simulink model "UNCCModel"  (R2018b)
settings: Solver=ode4  StartTime=0.0  StopTime=Inf  FixedStep=0.025  RelTol=1e-3  EnableMultiTasking=on
PreLoadFcn:
  | preLoadCallback
StartFcn:
  | startCallback
StopFcn:
  | stopCallback
model workspace (MAT data in the model file):
  Ts = 0.025
undefined symbols (not defined in the file or in its folder): acA2000, Ace, Basler, Freerun_FIX_YAW, PoCL
libraries: slrtlib x3, xpcbitflowlib x3, xpcvideoutillib x2, xpcobsoletelib x1, xpcrtudplib x1
(part 3 of 3)

== matlab function UNCCModel/cam3A/convertPixelsToCM ==
  data: d input; xx output; yx output; xTop input; xBottom input; yTop input; yBottom input; viewAngle input
function [xx,yx] = ...
    convertPixelsToLength(d,xTop,xBottom,yTop,yBottom,viewAngle)
%#codegen

% INPUTS:
% d - distance from camera to dot centroid
% xTop - horizontal pixel coordinate location of left dot in the frame
% xBottom - horizontal pixel coordinate location of the right dot in the
% frame
% yTop - vertical pixel coordinate location of the left dot in the frame
% yBottom -  vertical pixel coordinate location of the right dot in the
% frame
% viewAngle - two element vector, first characterizes the width of the
% field of view (camera horizontal), the second characterizes the height of
% the field of veiw (camera vertical).

% Calculate dot separations in pixels
% Camera-X separation will contribute to y component of body fixed x unit
% vector, if top dot is to the left of bottom dot (xTop<xBottom), then the component will
% have a negative value.  Camera-Y separation will contribute to x 
% component of body fixed x unit vector if top dot is above bottom dot 
% (yTop<yBottom), then this should have a positive value.  Note that 
% coordinate origin of pixels is in the upper left of the frame and the 
% positive y points down.
xx = -(yTop - yBottom);
yx =  (xTop - xBottom); 


% Convert pixels to length
% The (2*d*tand(viewAngle(1))) term calculates the total horizontal (or
% vertical)
% distance spanned by the camera field of view, the /2040 and /1080 terms
% normalize the separations by the total number of pixels.
xx = (2*d*tand(viewAngle(2)))*(xx/1088);
yx = (2*d*tand(viewAngle(1)))*(yx/2040);


xc=(yTop+yBottom)/2;
yc=(xTop+xBottom)/2;
xx = xx/cosd(20*((544-xc)/544));
yx = yx/cosd(20*((1020-yc)/1020));

== matlab function UNCCModel/cam2/convertPixelsToCM ==
  data: d input; yy output; zy output; xLeft input; xRight input; yLeft input; yRight input; viewAngle input
function [yy, zy] = ...
    convertPixelsToLength(d,xLeft,xRight,yLeft,yRight,viewAngle)
%#codegen

% INPUTS:
% d - distance from camera to dot centroid
% xLeft - horizontal pixel coordinate location of left dot in the frame
% xRight - horizontal pixel coordinate location of the right dot in the
% frame
% yLeft - vertical pixel coordinate location of the left dot in the frame
% yRight -  vertical pixel coordinate location of the right dot in the
% frame
% viewAngle - two element vector, first characterizes the width of the
% field of view (camera horizontal), the second characterizes the height of
% the field of veiw (camera vertical).

% Calculate dot separations in pixels
% Camera-X separation will contribute to y component of body fixed y unit
% vector, if left dot is to the left of right dot (xLeft<xRight), then the 
% component will have a positive value.  Camera-Y separation
% will contribute to z component of body fixed y unit vector if left dot is
% below right dot (yLeft>yRight),
% then this should have a positive value.
yy = -(xLeft - xRight); 
zy =  (yLeft - yRight);

% Convert pixels to length
% The (2*d*tand(viewAngle(1))) term calculates the total horizontal (or
% vertical)
% distance spanned by the camera field of view, the /2040 and /1080 terms
% normalize the separations by the total number of pixels.
yy = (2*d*tand(viewAngle(1)))*(yy/2040); % y component of body fixed y
zy = (2*d*tand(viewAngle(2)))*(zy/1088); % z component of body fixed y


yc=(xLeft+xRight)/2;
zc=(yLeft+yRight)/2;
yy = yy/cosd(20*((544-yc)/544));
zy = zy/cosd(20*((1020-zc)/1020));

== matlab function UNCCModel/cam3B/convertPixelsToCM ==
  data: d input; xy output; yy output; xLeft input; xRight input; yLeft input; yRight input; viewAngle input
function [xy, yy] = ...
    convertPixelsToLength(d,xLeft,xRight,yLeft,yRight,viewAngle)
%#codegen

% INPUTS:
% d - distance from camera to dot centroid
% xLeft - horizontal pixel coordinate location of left dot in the frame
% xRight - horizontal pixel coordinate location of the right dot in the
% frame
% yLeft - vertical pixel coordinate location of the left dot in the frame
% yRight -  vertical pixel coordinate location of the right dot in the
% frame
% viewAngle - two element vector, first characterizes the width of the
% field of view (camera horizontal), the second characterizes the height of
% the field of veiw (camera vertical).

% Calculate dot separations in pixels
% Camera-X separation will contribute to y component of body fixed y unit
% vector, if left dot is to the left of right dot (xLeft<xRight), then the 
% component will have a positive value.  Camera-Y separation
% will contribute to x component of body fixed y unit vector if left dot is
% below right dot (yLeft>yRight),
% then this should have a positive value.
yy = -(xLeft - xRight); 
xy =  (yLeft - yRight);

% Convert pixels to length
% The (2*d*tand(viewAngle(1))) term calculates the total horizontal (or
% vertical)
% distance spanned by the camera field of view, the /2040 and /1080 terms
% normalize the separations by the total number of pixels.
xy = (2*d*tand(viewAngle(1)))*(xy/2040); % y component of body fixed y
yy = (2*d*tand(viewAngle(2)))*(yy/1080); % z component of body fixed y


yc=(xLeft+xRight)/2;
xc=(yLeft+yRight)/2;
yy = yy/cosd(20*((544-yc)/544));
xy = xy/cosd(20*((1020-xc)/1020));

== matlab function UNCCModel/cam3A/convertAbsolutePositionToCM ==
  data: rCam input; xCam input; yCam input; viewAngle input; d input; r output
function r = convertAbsolutePositionsToCM(rCam, xCam, yCam,  viewAngle, d)
%#codegen
% This function calculates the x, y and z position of the dots in the
% ground fixed coordinates

% INPUTS
% rCam - 3 element vector of the camera position in the ground fixed frame
% units:cm
% xCam - horitontal location of the dots centroid in the image frame
% units:pixels
% yCam - vertical location of the dots centroid in the image frame
% units:pixels
% viewAngle - two element vector, first characterizes the width of the
% field of view (camera horizontal), the second characterizes the height of
% the field of veiw (camera vertical).
% d - distance from the camera to the dots

% Calculate the x and y locations
% If the horizontal location of the dots centroid in the image frame is
% to the left of the centerline (xCam<1020) then the y position of the dots
% centroid in the ground fixed frame will be greater than the y position of
% the camera in the ground fixed frame.
% If the vertical location of the dots centroid in the image frame is
% below the centerline (yCam>544) then the x position of the dots
% centroid in the ground fixed frame will be greater than the x position of
% the camera in the ground fixed frame.
% d=50;
x = rCam(1) + (yCam - 544 )*((2*d*tand(viewAngle(1)))/1088);
y = rCam(2) - (xCam - 1020)*((2*d*tand(viewAngle(2)))/2040);

% Calculate the z coordinate of the centroid of the dots.
% We know the x and y coordinate, the position of the camera, and the
% distance fromt the cammera to the dots.  Therfore, the solution is the
% value of z which causes the position to lie on the sphere centered on the
% camera with radius = d
z = 0;
% Check first to make sure that the value under the sqrt is positive
if d^2-(x - rCam(1))^2-(y - rCam(2))^2>=0
    z  = rCam(3) + sqrt(d^2-(x - rCam(1))^2-(y - rCam(2))^2);
end

r  =  [x y z];

== matlab function UNCCModel/cam3B/convertAbsolutePositionToCM ==
  data: rCam input; xCam input; yCam input; viewAngle input; d input; r output
function r = convertAbsolutePositionsToCM(rCam, xCam, yCam,  viewAngle, d)
%#codegen
% This function calculates the x, y and z position of the dots in the
% ground fixed coordinates

% INPUTS
% rCam - 3 element vector of the camera position in the ground fixed frame
% units:cm
% xCam - horitontal location of the dots centroid in the image frame
% units:pixels
% yCam - vertical location of the dots centroid in the image frame
% units:pixels
% viewAngle - two element vector, first characterizes the width of the
% field of view (camera horizontal), the second characterizes the height of
% the field of veiw (camera vertical).
% d - distance from the camera to the dots

% Calculate the x and y locations
% If the horizontal location of the dots centroid in the image frame is
% to the left of the centerline (xCam<1020) then the y position of the dots
% centroid in the ground fixed frame will be less than the y position of
% the camera in the ground fixed frame.
% If the vertical location of the dots centroid in the image frame is
% below the centerline (yCam>544) then the x position of the dots
% centroid in the ground fixed frame will be greater than the x position of
% the camera in the ground fixed frame.
% d=50;
x = rCam(1) + (yCam - 544 )*((2*d*tand(viewAngle(1)))/1088);
y = rCam(2) + (xCam - 1020)*((2*d*tand(viewAngle(2)))/2040);

% Calculate the z coordinate of the centroid of the dots.
% We know the x and y coordinate, the position of the camera, and the
% distance fromt the cammera to the dots.  Therfore, the solution is the
% value of z which causes the position to lie on the sphere centered on the
% camera with radius = d
z = 0;
% Check first to make sure that the value under the sqrt is positive
if d^2-(x - rCam(1))^2-(y - rCam(2))^2>=0
    z  = rCam(3) + sqrt(d^2-(x - rCam(1))^2-(y - rCam(2))^2);
end

r  =  [x y z];

== matlab function UNCCModel/MATLAB Function1 ==
  data: errorFlag input; controlMode input; motorVoltages output; closedLoopMotorCommands input; GUIMotorCommands input; saturation input
function motorVoltages = fcn(errorFlag,controlMode, closedLoopMotorCommands, GUIMotorCommands,saturation)
%#codegen

motorVoltages = GUIMotorCommands*1.65;
if controlMode == 1 % control mode 1 is closed loop control
    motorVoltages = closedLoopMotorCommands;
    
end

motorVoltages = motorVoltages + 1.65; %apply constant offset

if errorFlag ==1 % if there's a NaN error, zero all motors
    motorVoltages = 1.65*[1 1 1]';
    
end
for i = 1:3
    if motorVoltages(i)>saturation
        motorVoltages(i)=saturation;
    end
end

end

== matlab function UNCCModel/pitchDeadband ==
  data: onOff input; thetaSP input; theta input; error output; DBUpperLim input; DBLowerLim input
function error = fcn(onOff,thetaSP,theta,DBUpperLim,DBLowerLim)
%#codegen
error = 0;
if onOff == 1 % if onOff = 1, turn on the deadband
    if theta < thetaSP + DBLowerLim
        error = DBLowerLim - theta;
    end
    
    if theta > thetaSP + DBUpperLim
        error = DBUpperLim - theta;
    end
else % if onOff !=0 then turn off the deadband and use normal error
    error = thetaSP-theta;
end
end

== matlab function UNCCModel/cam1/Dot_detector_pitch ==
  data: uOut output; u input; roiDims input; locationMethod input; dotConfig input; centroidOverrideCommand input; rCentroidManualOverride input; clusteringParameters input; rCentroidAuto input; r1Img output; r2Img output; rCentroidImg output; viewOptions input
function [uOut,r1Img,r2Img,rCentroidImg] =...
    dotFinder(u,roiDims, locationMethod, dotConfig,centroidOverrideCommand,rCentroidManualOverride,clusteringParameters,rCentroidAuto,viewOptions)
%#codegen
% EXPLANATION OF INPUTS
% u = source image
% roiDims = 4 by 1 vector containing ROI dimensions
% locationMethod = 0 for centroid based dot location
% locationMethod = 1 for cluster based dot location (longer runtime but
% more robust
% dotConfig = 0 for horizontally arranged dots
% dotConfig = 1 for vertically arranged dots
% centroidOverrideCommand = 0 for automatic movemennt of ROI
% centroidOverrideCommand = 1 to use user input as ROI location
% rCentroidManualOverride: 2 element vector where element 1 is x or column
% of ROI centroid and element 2 is y or row of ROI, both of which are
% manually enetered by used
% rCentroidAuto: 2 element vector where element 1 is x or column of ROI
% centroid and element 2 is y or row of ROI, both of which are
% automatically generated from previous iteration
% viewOptions : 8 element vector where each element is a binary on/off
% switch to a certain part of the output view window
%
% WHAT THIS CODE IS
% Method : Centroid Only
%
% This code is a first attempt at rewriting the code to allow for adaptable
% implemmentation.
% Adaptable implemmentation will ultimately include:
% switch to change between DB clustering and centroid method
%



%%%%%%%%%%%%%%%%%%%%
% SET ROI DIMENSIONS
%%%%%%%%%%%%%%%%%%%%
[ roiHalfwidth, roiHalfheight ] = getROIDimensions(dotConfig,roiDims,centroidOverrideCommand);

%%%%%%%%%%%%%%%%%%%%
% PARSE INPUTS
%%%%%%%%%%%%%%%%%%%%

[dotConfig, locationMethod, centroidOverrideCommand ,rCentroidManualOverride ,viewOptions,roiHalfwidth, roiHalfheight]...
    =parseInputs(dotConfig, locationMethod, centroidOverrideCommand ,rCentroidManualOverride ,viewOptions,roiHalfwidth, roiHalfheight);

%%%%%%%%%%%%%%%%%%%%
%%SET ROI LOCATION%%
%%%%%%%%%%%%%%%%%%%%
rCentroid = rCentroidAuto;
if centroidOverrideCommand == 1  %Override with user input if commanded to do so
    rCentroid = rCentroidManualOverride;
end

%%%%%%%%%%%%%%%%%%%%%%%%%%%%%%%%%%%%
% EXTRACT ROI FROM ORIGIONAL IMAGE %
%%%%%%%%%%%%%%%%%%%%%%%%%%%%%%%%%%%%
roi=u(rCentroid(2) - roiHalfheight : rCentroid(2) + roiHalfheight , rCentroid(1) - roiHalfwidth : rCentroid(1) + roiHalfwidth);

%%%%%%%%%%%%%%%%%%%%%%%%%%%%%
%%%%OTSUS METHOD THRESHOLDING
%%%%%%%%%%%%%%%%%%%%%%%%%%%%%
roi=threshold(roi);


%%%%%%%%%%%%%%%%
% DOT LOCATION %
%%%%%%%%%%%%%%%%
%Preallocate to avoid "Variable undefined on some iteration paths" compile
%error
r1ROI        = [0,0]; r2ROI        = [0,0]; rCentroidROI = [0,0];
if locationMethod == 0; %USE CENTROID BASED METHOD
    if dotConfig == 0 %%HORIZONTAL DOTS
        [r1ROI,r2ROI,rCentroidROI] = centroidMethodHorizontal(roi,roiHalfwidth,roiHalfheight);
    else                %%VERTICAL DOTS
        [r1ROI,r2ROI,rCentroidROI] = centroidMethodVertical(roi,roiHalfwidth,roiHalfheight);
    end
else %USE CLUSTERING BASED METHOD (NOT CURRENTLY IMPLEMENTED)
    %%%REPLACE THIS CODE WITH CLUSTERING METHOD WHEN IMPLEMENTING
    %%%UNCOMMENT CODE BELOW ONCE clusterMethod FUNCTION IS WRITTEN
    %%%[r1ROI,r2ROI,rCentroidROI] = clusterMethod(roi,clusteringParameters);
    if dotConfig == 0 %%HORIZONTAL DOTS
        [r1ROI,r2ROI,rCentroidROI] = centroidMethodHorizontal(roi,roiHalfwidth,roiHalfheight);
    else                %%VERTICAL DOTS
        [r1ROI,r2ROI,rCentroidROI] = centroidMethodVertical(roi,roiHalfwidth,roiHalfheight);
    end
end
%%%%%%%%%%%%%%%%%%%%%%%%%
%%%%PARSE DOT LOCATIONS %
%%%%%%%%%%%%%%%%%%%%%%%%%
%IF DOT CENTER LOCATION ALGORITHM HAS FAILED (OUTPUT = NONSENSE) THEN
%OVERRIDE CENTROID COORDINATES WITH DEFAULT VALUES TO PREVENT PROBLEMS
%LATER
[r1ROI,r2ROI,rCentroidROI] = parseDotLocations(dotConfig,r1ROI,r2ROI,rCentroidROI,roiHalfwidth,roiHalfheight);

%%%%%%%%%%%%%%%%%%%%%%%%%%%%%%%%%%%%%%%%%%%%%%%%%%%
%%%%TRANSFORM BACK TO ORIGIONAL IMAGE COORDINATES %
%%%%%%%%%%%%%%%%%%%%%%%%%%%%%%%%%%%%%%%%%%%%%%%%%%%
%Preallocate to avoid "Variable undefined on some iteration paths" compile
%error
r1Img         = [0,0]; r2Img         = [0,0]; rCenntroidImg = [0,0];

if dotConfig == 0  %HORIZONTALLY ARRANGED DOTS
    [r1Img, r2Img, rCentroidImg] = convertCoordinatesHorizontal(r1ROI,r2ROI,rCentroid,roiHalfwidth,roiHalfheight);
else % VERTICALLY ARRANGED DOTS
    [r1Img, r2Img, rCentroidImg] = convertCoordinatesVertical(r1ROI,r2ROI,rCentroid,roiHalfwidth,roiHalfheight);
end
%%%%%%%%%%%%%%%%%%%%%
% DRAW OUTPUT IMAGE %
%%%%%%%%%%%%%%%%%%%%%

uOut  =  drawOutputImage(viewOptions,u,roi,r1Img,r2Img,rCentroid,r1ROI,r2ROI,roiHalfwidth,roiHalfheight);


end



%DRAW OUTPUT IMAGE
function uOut  =  drawOutputImage(viewOptions,uOut,roi,r1Img,r2Img,rCentroid,r1ROI,r2ROI,roiHalfwidth,roiHalfheight)
%function takes the origional image "u" and redraws it as the output image
%uOut
%View options 7 and 8 are currently not used, can/will be used later for
%clustering algorithm outputs
if viewOptions(1) == 1 %View option = draw any features on output view at all
    if viewOptions(2) == 1 %Draw Features in main image
        if viewOptions(3) == 1 %Draw ROI box in main image
            uOut(rCentroid(2) - roiHalfheight : rCentroid(2) + roiHalfheight, rCentroid(1) - roiHalfwidth                               )=255; %Draw left edge of roi box
            uOut(rCentroid(2) - roiHalfheight : rCentroid(2) + roiHalfheight, rCentroid(1) + roiHalfwidth                               )=255; %Draw right edge of roi box
            uOut(rCentroid(2) - roiHalfheight                               , rCentroid(1) - roiHalfwidth : rCentroid(1)+roiHalfwidth  )=255; %Draw top edge of roi box
            uOut(rCentroid(2) + roiHalfheight                               , rCentroid(1) - roiHalfwidth : rCentroid(1)+roiHalfwidth  )=255; %Draw bottom edge of roi box
        end
        if viewOptions(4) == 1 %Draw crosshairs in main image
            uOut(: ,r1Img(1)  ) = 255;
            uOut(: ,r2Img(1) ) = 255;
            uOut(r1Img(2) ,:  ) = 255;
            uOut(r2Img(2),:  ) = 255;
        end
    end
    if viewOptions(5) == 1 %Draw thresholding in lower left
        roi = 255*roi;
        if viewOptions(6) == 1% Draw crosshairs on thresholding
            roi(r1ROI(2) , :           ) = 255;
            roi(r2ROI(2), :           ) = 255;
            roi(:           , r1ROI(1) ) = 255;
            roi(:           , r2ROI(1)) = 255;
        end
        uOut (1080-size(roi,1)+1:1080, 1:size(roi,2)) = roi;
    end
end
end

%CONVERT ROI COORDINATES TO IMG COORDINATES (HORIZONTAL)
function [rLeftImg, rRightImg, rCentroidImg] = convertCoordinatesHorizontal(rLeftROI,rRightROI,rCentroid,roiHalfwidth,roiHalfheight)
%This function takes in the dot positions in the ROI frame of reference
%and outputs coordinates in the origional image frame of reference, all in
%vectorize format [x,y].  Note that x = column and y = row.

%Convert y (row) coordinates
yLImg = rCentroid(2) - roiHalfheight + rLeftROI(2);
yRImg = rCentroid(2) - roiHalfheight + rRightROI(2);
%Convert x (col) coordinates
xLImg = rCentroid(1) - roiHalfwidth + rLeftROI(1);
xRImg = rCentroid(1) - roiHalfwidth + rRightROI(1);
%Put results into vector format
rLeftImg  = [ xLImg, yLImg ];
rRightImg = [ xRImg, yRImg ];
%Calculate ROI cenntroid as average of two dot coordinates
rCentroidImg = [fix((xLImg+xRImg)/2),fix((yLImg+yRImg)/2)];

end

%CONVERT ROI COORDINATES TO IMG COORDINATES (VERTICAL)
function [rTopImg, rBottomImg, rCentroidImg] = convertCoordinatesVertical(rTopROI,rBottomROI,rCentroid,roiHalfwidth,roiHalfheight)
%This function takes in the dot positions in the ROI frame of reference
%and outputs coordinates in the origional image frame of reference, all in
%vectorize format [x,y].  Note that x = column and y = row.

%Convert y (row) coordinates
yTImg = rCentroid(2) - roiHalfheight + rTopROI(2);
yBImg = rCentroid(2) - roiHalfheight + rBottomROI(2);
%Convert x (col) coordinates
xTImg = rCentroid(1) - roiHalfwidth + rTopROI(1);
xBImg = rCentroid(1) - roiHalfwidth + rBottomROI(1);
%Put results into vector format
rTopImg    = [ xTImg, yTImg ];
rBottomImg = [ xBImg, yBImg ];
%Calculate ROI cenntroid as average of two dot coordinates
rCentroidImg = [fix((xTImg+xBImg)/2),fix((yTImg+yBImg)/2)];

end

%CENTROID METHOD DOT LOCATION (HORIZONTAL)
function [rLeft,rRight,rCentroid] = centroidMethodHorizontal(roi,roiHalfwidth,roiHalfheight)
%Function returns the position of the dots rCentroid as well as the
%centroid of the overall image rCentroid
%Calculated by using centroid method, assuming the dots are arranged
%horizontally

%Divide the image in half vertically (left and right)
roiLeft  = roi( : , 1            : roiHalfwidth);
roiRight = roi( : , roiHalfwidth : end         );

%Calculate the x coordinates of the centroids
xLROI = round(sum((sum(roiLeft ,1) .* (1:size(roiLeft ,2))))/sum(sum(roiLeft )));
xRROI = round(sum((sum(roiRight,1) .* (1:size(roiRight,2))))/sum(sum(roiRight)))+roiHalfwidth;
%Calculate the y coordinates of the centroids
yLROI = round(sum((sum(roiLeft ,2) .* (1:size(roiLeft, 1))'))/sum(sum(roiLeft )));
yRROI = round(sum((sum(roiRight,2) .* (1:size(roiRight,1))'))/sum(sum(roiRight)));
%Put results into vector format
rLeft     = [xLROI, yLROI];
rRight    = [xRROI, yRROI];
%Find ROI cenntroid as the average position of the two centroids
rCentroid = [fix((xLROI+xRROI)/2),fix((yLROI+yRROI)/2)];
end

%CENTROID METHOD DOT LOCATION (VERTICAL)
function [rTop,rBottom,rCentroid] = centroidMethodVertical(roi,roiHalfwidth,roiHalfheight)
%Function returns the position of the dots rCentroid as well as the
%centroid of the overall image rCentroid
%Calculated by using centroid method assuming the dots are arranged
%vertically;

%Divide the image in half horizontally (top and bottom)
roiTop    = roi( 1             : roiHalfheight , : );
roiBottom = roi( roiHalfheight : end           , : );

%Calculate the x coordinates of the centroids
xTROI = round(sum((sum(roiTop   ,1) .* (1:size(roiTop   ,2))))/sum(sum(roiTop )));
xBROI = round(sum((sum(roiBottom,1) .* (1:size(roiBottom,2))))/sum(sum(roiBottom)));

%Calculate the y coordinates of the centroids
yTROI = round(sum((sum(roiTop   ,2) .* (1:size(roiTop   ,1))'))/sum(sum(roiTop )));
yBROI = round(sum((sum(roiBottom,2) .* (1:size(roiBottom,1))'))/sum(sum(roiBottom)))+roiHalfheight;
%Put results into vector format
rTop     = [xTROI, yTROI];
rBottom  = [xBROI, yBROI];
%Find ROI cenntroid as the average position of the two centroids
rCentroid = [fix((xTROI+xBROI)/2),fix((yTROI+yBROI)/2)];
end

%CLUSTERING METHOD DOT LOCATION
function [rTop,rBottom,rCentroid] = clusterMethod(roi,clusteringParameters)
%This function is currently a placeholder, will be used later if/when
%clustering is implemented
end

%IMAGE THRESHOLDING - OTSU'S METHOD
function img = threshold(img)
%This function takes in a grayscale matrix and outputs a thresholded,
%binaray matrix according to Otsus Method.

%Generate histogram of image
counts=zeros(256,1);
[m,n]=size(img);
for i = 1:m*n
    counts(img(i)+1)=counts(img(i)+1)+1;
end
%Callculate variances
p = counts / sum(counts);
sigma_b=zeros(256,1);
%%%%%%%%%%%%%%%%55
%POSSIBLE DIV BY ZERO ERRORS HERE?
%%%%%%%%%%%%%%%%%%%%%%
for t = 1 : 256
    q_L = sum(p(1 : t));
    q_H = sum(p(t + 1 : end));
    miu_L = sum(p(1 : t) .* (1 : t)') / q_L;
    miu_H = sum(p(t + 1 : end) .* (t + 1 : 256)') / q_H;
    sigma_b(t) = q_L * q_H * (miu_L - miu_H)^2;
end
% Desired threshold is the max of sigma_b vector
[~,threshold_otsu] = max(sigma_b(:));
% Threshold image as those points above the threshold value
img=(img>threshold_otsu);
end

%INPUT PARSING
function        [dotConfig, locationMethod, centroidOverrideCommand ,rCentroidManualOverride ,viewOptions,roiHalfwidth, roiHalfheight]...
    =parseInputs(dotConfig, locationMethod, centroidOverrideCommand ,rCentroidManualOverride ,viewOptions,roiHalfwidth, roiHalfheight)
% This function parses inputs and corrects potentially harmful/unstable
% inputs.
locationMethod            = setToBinary(locationMethod);
centroidOverrideCommand   = setToBinary(centroidOverrideCommand);

if centroidOverrideCommand == 1
    if numel(rCentroidManualOverride)~=2
        rCentroidManualOverride = [540,1020];
    end
    if rCentroidManualOverride(2) > 1080 - roiHalfheight - 1
        rCentroidManualOverride(2) = 1080 - roiHalfheight - 1;
    end
    if rCentroidManualOverride(1) > 2040 - roiHalfwidth - 1
        rCentroidManualOverride(1) = 2040 - roiHalfwidth - 1;
    end
    
    if rCentroidManualOverride(2) < roiHalfheight + 1
        rCentroidManualOverride(2) = roiHalfheight + 1;
    end
    if rCentroidManualOverride(1) < roiHalfwidth + 1
        rCentroidManualOverride(1) = roiHalfwidth + 1;
    end
    
    
end

if numel(viewOptions) > 8
    viewOptions = viewOptions(1:8);
end
if numel(viewOptions) < 8
    viewOptions = [0,0,0,0,0,0,0,0];
end
for i=1:8
    viewOptions(i) = setToBinary(viewOptions(i));
end
rCentroidManualOverride=fix(rCentroidManualOverride);
dotConfig = setToBinary(dotConfig);

end

%ROUND TO BINARY VALUE
function [out] = setToBinary(in)
%takes any numerical input and sets it to either 0 or 1 depending on
%what's closer
out = in;
if out>1
    out=1;
end
if out<0
    out=0;
end
if out >0  && out <1
    out=round(out);
end
end

%GET ROI DIMENSIONS
function [roiHalfwidth,roiHalfheight] = getROIDimensions(dotConfig,roiDims,centroidOverrideCommand)
%This function sets the ROI Dimensions depending on user input
%(dotConfig).


if numel(roiDims)==5 %Check to make sure ROI dimension vector is right length
    for i = 1 : 4   %Saturation, make sure roi dimension vector elements make sense, if not set them to something more reasonable
        if roiDims(i)>500
            roiDims(i)=500;
        end
        
        if roiDims(i)<20
            roiDims(i)=20;
        end
    end
%     if centroidOverrideCommand == 0
%         for i = 1:4
%             roiDims(i) = roiDims(1)+roiDims(i)*((d-(50-rCam(2)))/50)*roiDims(5);
%         end
%     end
    
    
    if dotConfig == 1 %VERTICAL ARRANGEMENT
        roiHalfwidth = roiDims(1);
        roiHalfheight = roiDims(2);
        
    else
        roiHalfwidth = roiDims(3);
        roiHalfheight = roiDims(4);
    end
end

end

%PARSE DOT LOCATIONS
function [r1ROI,r2ROI,rCentroidROI] = parseDotLocations(dotConfig,r1ROI,r2ROI,rCentroidROI,roiHalfwidth,roiHalfheight)
if dotConfig == 0 %HORIZONTAL DOTS
    if isnan(r1ROI(1))
        r1ROI(1)=fix(roiHalfwidth/2);
    end
    if isnan(r1ROI(2))
        r1ROI(2)=roiHalfheight;
    end
    if isnan(r2ROI(1))
        r2ROI(1)=fix(3*roiHalfheight/2);
    end
    if isnan(r2ROI(2))
        r2ROI(2)=roiHalfheight;
    end
else %VERTICAL DOTS
    if isnan(r1ROI(1))
        r1ROI(1)=roiHalfwidth;
    end
    if isnan(r1ROI(2))
        r1ROI(2)=fix(roiHalfheight/2);
    end
    if isnan(r2ROI(1))
        r2ROI(1)=roiHalfwidth;
    end
    if isnan(r2ROI(2))
        r2ROI(2)=fix(3*roiHalfheight/2);
    end
end

if isnan(rCentroidROI(1))
    rCentroidROI(1)=roiHalfwidth;
end

if isnan(rCentroidROI(2))
    rCentroidROI(2) = roiHalfheight;
end


end

== matlab function UNCCModel/altitudeDeadband ==
  data: onOff input; zSP input; z input; error output; DBUpperLim input; DBLowerLim input
function error = deadband(onOff,zSP,z,DBUpperLim,DBLowerLim)
%#codegen
error = 0;
if onOff == 1 % if onOff = 1, turn on the deadband
    if z < zSP + DBLowerLim
        error = DBLowerLim - z;
    end
    
    if z > zSP + DBUpperLim
        error = DBUpperLim - z;
    end
else % if onOff !=0 then turn off the deadband and use normal error
    error = zSP-z;
end
end

== matlab function UNCCModel/findUnitVectors ==
  data: xxCam1 input; rx output; xxCam3a input; yxCam3a input; zxCam1 input; ry output; rz output; error output; xyCam3b input; yyCam2 input; yyCam3b input; zyCam2 input; sideSep input; bottomASep input; bottomBSep input; cameraAngle input
function [rx,ry,rz,error] = findUnitVectors(xxCam1,xxCam3a,yxCam3a,zxCam1,...
    xyCam3b,yyCam2,yyCam3b,zyCam2,sideSep,bottomASep,bottomBSep,cameraAngle)
%#codegen

% This function has 2 purposes:
% 1) Resolve components of the body fixed unit vectors in the
% ground fixed coordinate system
% 2) Calculate a signal which characterizes how successful the orientation
% resolution is. It does this by computing the dot product of the 
% normalized body fixed x unit vector and the normalized body fixed y unit 
% vector.  The result is output as the "error".  In a perfect system, this
% value would always be zero.


% The z component of the y unit vector (zyCam2) be effected by the angle of
% the camera, as well as the yaw.
% Note that cam 2 and cam 3b are tracking the same dots so no need to
% normalize before this calculation.
zyCam2 = (zyCam2-xyCam3b*sind(cameraAngle))/cosd(cameraAngle);
yyCam2 = (yyCam2-xyCam3b*cosd(cameraAngle))/sind(cameraAngle);
% note that the x component of the x unit vector and the y component of the
% y unit vector are both over-determined (calculated twice).  We're gonna
% use this to our advantage by constructing the x and y unit vectors twice
% and then taking their average.  Hopefully this will smooth out some
% noise and reduce error somewhat.

% Calculate the body fixed x unit vectors
rx1 = [xxCam1  yxCam3a*sideSep/bottomASep zxCam1];
rx2 = [xxCam3a yxCam3a                    zxCam1*bottomASep/sideSep];

% normalize both vectors
rx1 = rx1./sqrt((rx1(1))^2+(rx1(2))^2+(rx1(3))^2);
rx2 = rx2./sqrt((rx2(1))^2+(rx2(2))^2+(rx2(3))^2);

% average the two vectors
rx = (rx1+rx2)./2;

% normalize the result
rx = rx./sqrt((rx(1))^2+(rx(2))^2+(rx(3))^2);

% Calculate the body fixed y unit vectors
ry1 = [xyCam3b yyCam2 zyCam2];  % This line seems
% problematic, probably need to do an adjustment to yyCam2 before
% implementing this.  Similiar to adjustment done to zyCam2 above.
% ry = [xyCam3b                       yyCam3b zyCam2*bottomASep/bottomBSep];
ry2 = [xyCam3b yyCam3b zyCam2]; % cam3b and cam2 track the same dots, so there should be no need for scaling/normalization in this line


% normalize both vectors
ry1 = ry1./sqrt((ry1(1))^2+(ry1(2))^2+(ry1(3))^2);
ry2 = ry2./sqrt((ry2(1))^2+(ry2(2))^2+(ry2(3))^2);

% average the two vectors
ry = (ry1+ry2)./2;

% normalize the result
ry = ry./sqrt((ry(1))^2+(ry(2))^2+(ry(3))^2);

% z = x cross y
rz = cross(rx, ry);

% error is the dot product of the two
error = dot(rx,ry);
end

== matlab function UNCCModel/findEulerAngles ==
  data: rx input; ry input; rz input; roll output; pitch output; yaw output; R output
function [roll,pitch,yaw,R] = findEulerAngles(rx,ry,rz)
%#codegen
% The purpose of this function is to calculate the euler angles from the
% body fixed unit vectors rx, ry and rz.

% Build rotation matrix from unit vectors, spell it out explicitly for
% safety since I don't know if rx, ry and rz are being passed as row or
% column vectors
% R is rotation matrix from body fixed coordinates to ground fixed
% coordinates
R = [rx(1) ry(1) rz(1);...
     rx(2) ry(2) rz(2);...
     rx(3) ry(3) rz(3)];
 
 
 pitch = asin(-R(3,1));
 
 % Saturate the pitch to +/- pi/4 to avoid divide by zero errors in the
 % next step.
 if pitch > pi/4
     pitch = pi/4;
 end
 if pitch < -pi/4
     pitch = -pi/4;
 end
 % Note: arcsin gives a real answer on the range -1 to 1 so we should
 % saturate the argument to the arcsin function.
 
 yawArg = R(2,1)/cos(pitch);
 rollArg = R(3,2)/cos(pitch);
 
 if yawArg>1
     yawArg=1;
 end
 if yawArg<-1 
     yawArg=-1;
 end
 
  if rollArg>1
     rollArg=1;
 end
 if rollArg<-1 
     rollArg=-1;
 end
 
 yaw   = asin(yawArg);
 roll  = asin(rollArg);
 
end

== matlab function UNCCModel/cam1/MATLAB Function ==
  data: r_cam input; d_cam_com output; r_com input; x_dist output; y_dist output; z_dist output
function [d_cam_com , x_dist, y_dist, z_dist] = distanceToCenterOfMass(r_cam , r_com)
%Function exists to calculate the distance between the camera and the
%center of mass in units of length
%#codegen

x_dist = abs(r_cam(1) - r_com(1));
y_dist = abs(r_cam(2) - r_com(2));
z_dist = abs(r_cam(3) - r_com(3));

d_cam_com = ( x_dist^2 + y_dist^2 + z_dist^2 )^(1/2);

== matlab function UNCCModel/cam1/convertPixelsToCM ==
  data: d input; xx output; zx output; xLeft input; xRight input; yLeft input; yRight input; viewAngle input
function [xx, zx] = ...
    convertPixelsToLength(d,xLeft,xRight,yLeft,yRight,viewAngle)
%#codegen

% INPUTS:
% d - distance from camera to dot centroid
% xLeft - horizontal pixel coordinate location of left dot in the frame
% xRight - horizontal pixel coordinate location of the right dot in the
% frame
% yLeft - vertical pixel coordinate location of the left dot in the frame
% yRight -  vertical pixel coordinate location of the right dot in the
% frame
% viewAngle - two element vector, first characterizes the width of the
% field of view (camera horizontal), the second characterizes the height of
% the field of veiw (camera vertical).

% Calculate dot separations in pixels
% Camera-X separation will contribute to x component of body fixed x unit
% vector, if left dot is to the left of right dot (xLeft<xRight), then the 
% component will have a positive value.  Camera-Y separation
% will contribute to z component of body fixed x unit vector if left dot is
% below right dot (yLeft>yRight),
% then this should have a positive value.
xx = -(xLeft - xRight); 
zx =  (yLeft - yRight);

% Convert pixels to length
% The (2*d*tand(viewAngle(1))) term calculates the total horizontal (or
% vertical)
% distance spanned by the camera field of view, the /2040 and /1080 terms
% normalize the separations by the total number of pixels.
xx = (2*d*tand(viewAngle(1)))*(xx/2040); % y component of body fixed y
zx = (2*d*tand(viewAngle(2)))*(zx/1088); % z component of body fixed y

xc=(xLeft+xRight)/2;
zc=(yLeft+yRight)/2;
xx = xx/cosd(20*((544-xc)/544));
zx = zx/cosd(20*((1020-zc)/1020));

== matlab function UNCCModel/cam1/convertAbsolutePositionToCM ==
  data: rCam input; xCam input; yCam input; viewAngle input; d input; r output
function r = convertAbsolutePositionsToCM(rCam, xCam, yCam,  viewAngle, d)
%#codegen
% This function calculates the x, y and z position of the dots in the
% ground fixed coordinates, r
% INPUTS
% rCam - 3 element vector of the camera position in the ground fixed frame
% units:cm
% xCam - horitontal location of the dots centroid in the image frame
% units:pixels
% yCam - vertical location of the dots centroid in the image frame
% units:pixels
% viewAngle - two element vector, first characterizes the width of the
% field of view (camera horizontal), the second characterizes the height of
% the field of veiw (camera vertical).
% d - distance from the camera to the dots
% Calculate the x and z locations
% If the horizontal location of the dots centroid in the image frame is
% to the left of the centerline (xCam<1040) then the x position of the dots
% centroid in the ground fixed frame will be less than the x position of
% the camera in the ground fixed frame.
% If the vertical location of the dots centroid in the image frame is
% below the centerline (yCam>544) then the z position of the dots
% centroid in the ground fixed frame will be less than the z position of
% the camera in the ground fixed frame.
% d=50;
x = rCam(1) + (xCam - 1020)*((2*d*tand(viewAngle(1)))/2040);
z = rCam(3) - (yCam - 544  )*((2*d*tand(viewAngle(2)))/1088);
% Calculate the y coordinate of the centroid of the dots.
% We know the x and z coordinate, the position of the camera, and the
% distance from the cammera to the dots.  Therfore, the solution is the
% value of y which causes the position to lie on the sphere centered on the
% camera with radius = d
y = 0;
% Check first to make sure that the value under the sqrt is positive
if d^2-(x - rCam(1))^2-(z - rCam(3))^2>=0
    y  = rCam(2) + sqrt(d^2-(x - rCam(1))^2-(z - rCam(3))^2); %rCam(2) should be very negative ~-50+ cm
end
r  =  [x y z];
